simulink model "movementCueEast"  (R2012b)
settings: Solver=FixedStepDiscrete  SolverMode=SingleTasking  StartTime=0.0  StopTime=inf  RelTol=1e-3
model workspace (MAT data in the model file):
  Param = Simulink.Parameter
  Param.DataType = 'auto'
undefined symbols (not defined in the file or in its folder): blockNumber, expRandBinSize, expRandMax, expRandMin, expRandMu, holdDuration, macaddr, modelConstants, movementDuration, pause, randomSeed, repsPerBlock, restDuration, returnDuration, useRandomDelay, whichMovements
libraries: xpcethernetlib x13, Lib_FileLogger x9, xpcnetworkbufferlib x4, xpclib x3, dspmtrx3 x2, xpcparallelportlib x1, simulink x1, Lib_CerebusRead x1
settings Model: xpc_rtwmakecfg_data=_xpcetherlib__xpcether8255xlib__xpcetherGbElib__xpcnblib_  Creator=gilja  LastModifiedBy=NPTL
settings OptimizationCC: BlockReduction=off  InlineParams=on  InlineInvariantSignals=on  SimCompilerOptimization=On
settings HardwareCC: ProdIntDivRoundTo=Zero  ProdEndianess=LittleEndian  ProdHWDeviceType=Generic->32-bit x86 compatible
settings RTWCC: SystemTargetFile=xpctarget.tlc  TemplateMakefile=xpc_default_tmf  Description=xPC Target  ProcessScript=xpctarget_make_rtw_hook  RTWCompilerOptimization=On
settings CodeAppCC: MaxIdLength=62
settings xpcTargetCC: TargetFcnLib=ansi_tfl_table_tmw.mat  CodeReplacementLibrary=XPC_BLAS  ParMdlRefBuildCompliant=on  ConcurrentExecutionCompliant=on  CombineSignalStateStructs=off  GRTInterface=on  xPCTaskExecutionProfile=off  xPCRL32EventNumber=5000  RL32IRQSourceModifier=5  xPCIRQSourceBoard=Parallel_Port  xPCIOIRQSlot=0x378  xPCisDownloadable=off  xPCLoadParamSetFile=off  xPCConcurrentTasks=off  xPCEnableSFAnimation=off

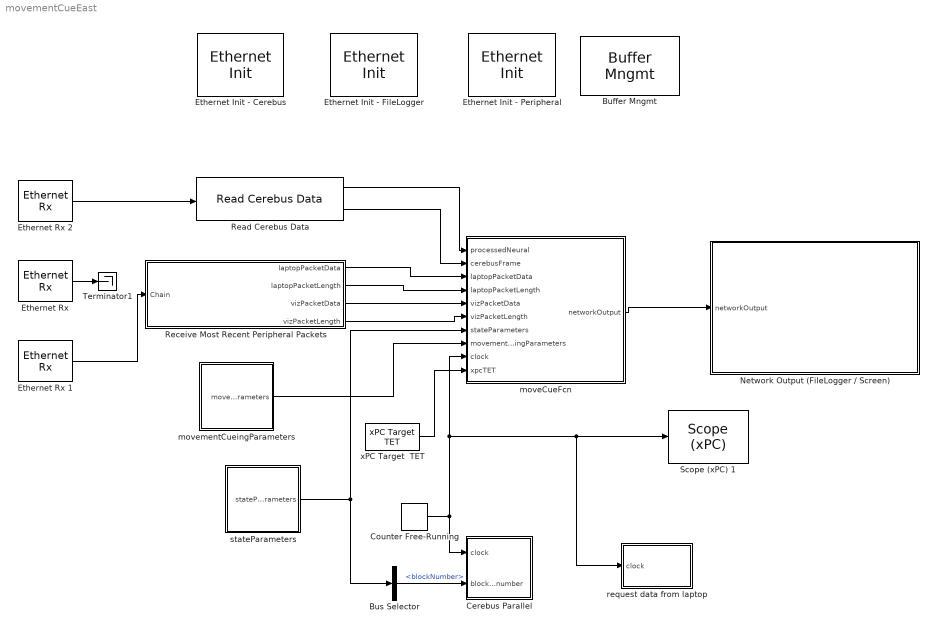
== system movementCueEast ==
  "Buffer Mngmt " : xpcnetworkbufferlib/Buffer Mngmt   Priority=-1  SampleTime=-1  PoolSizes=[100 10 10 200]  ShowTune=on
  Bus Selector : BusSelector  OutputSignals=blockNumber
  Cerebus Parallel : Subsystem
  Counter Free-Running : simulink/Sources/Counter Free-Running  NumBits=32  tsamp=-1
  Ethernet Init - Cerebus : xpcethernetlib/Ethernet Init   Priority=-1  ID=1  Driver=Intel Gigabit  Bus=3  Slot=14  SampleTime=-1  AddressSource=Specify  MAC=macaddr('00:00:00:00:00:00')  TxSA=off  RxPromiscuous=off  Multicast={}  RxBad=off  RxShort=off  MaxMTU=1518  TxThreshold=10  TxBuffers=128  RxBuffers=64  ShowTune=on  NumRxBlks=1
  Ethernet Init - FileLogger : xpcethernetlib/Ethernet Init   Priority=-1  ID=2  Driver=Intel Gigabit  Bus=3  Slot=13  SampleTime=-1  AddressSource=Specify  MAC=macaddr('00:00:00:00:00:00')  TxSA=off  RxPromiscuous=off  Multicast={}  RxBad=off  RxShort=off  MaxMTU=1518  TxThreshold=10  TxBuffers=128  RxBuffers=8  ShowTune=on  NumRxBlks=1
  Ethernet Init - Peripheral : xpcethernetlib/Ethernet Init   Priority=-1  ID=3  Driver=Intel Gigabit  Bus=2  Slot=0  SampleTime=-1  AddressSource=Specify  MAC=macaddr('00:00:00:00:00:00')  TxSA=off  RxPromiscuous=off  Multicast={}  RxBad=off  RxShort=off  MaxMTU=1518  TxThreshold=10  TxBuffers=128  RxBuffers=8  ShowTune=on  NumRxBlks=1
  "Ethernet Rx " : xpcethernetlib/Ethernet Rx   ID=2  SampleTime=modelConstants.sampleTime  Criteria=Receive all unmatched types [0 to 65535]  EtherType=[hex2dec('0000')]  BlkID=0
  Ethernet Rx 1 : xpcethernetlib/Ethernet Rx   ID=3  SampleTime=modelConstants.sampleTime  Criteria=Receive all unmatched types [0 to 65535]  EtherType=[hex2dec('0000')]  BlkID=0
  Ethernet Rx 2 : xpcethernetlib/Ethernet Rx   ID=1  SampleTime=modelConstants.sampleTime  Criteria=Receive all unmatched types [0 to 65535]  EtherType=[hex2dec('0000')]  BlkID=0
  Network Output (FileLogger / Screen) : Subsystem
  Read Cerebus Data : Lib_CerebusRead/Read Cerebus Data
  Receive Most Recent Peripheral Packets : Subsystem
  Scope (xPC) 1 : xpclib/Misc./Scope (xPC)   scopeno=1  scopetype=Target  autostart=on  viewmode=Numerical  formatstr='%15.6f'  grid=on  ylimits=[0,0]  nosamples=250  noprepostsamples=0  interleave=1  triggermode=FreeRun  triggersignal=1  triggerlevel=0.0  triggerslope=Either  triggerscope=1  triggersample=0  filename=data.dat  mode=Lazy  writesize=512  autorestart=off  dynamicfilemode=off  maxwritefilesize=512*1024^2
  Terminator1 : Terminator
  moveCueFcn : MATLAB Function  TreatAsAtomicUnit=on
  movementCueingParameters : Subsystem
  request data from laptop : Subsystem
  stateParameters : Subsystem
  "xPC Target  TET " : xpclib/Misc./xPC Target  TET   ts=0.001
  wires:
  Ethernet Rx 1/1 -> Receive Most Recent Peripheral Packets/1(Chain)
  moveCueFcn/1(networkOutput) -> Network Output (FileLogger / Screen)/1(networkOutput)
  stateParameters/1(stateParameters) -> Bus Selector/1, moveCueFcn/7(stateParameters)
  "Ethernet Rx "/1 -> Terminator1/1
  Counter Free-Running/1 -> Scope (xPC) 1/1, request data from laptop/1(clock), moveCueFcn/9(clock), Cerebus Parallel/1(clock)
  movementCueingParameters/1(movementCueingParameters) -> moveCueFcn/8(movementCueingParameters)
  Bus Selector/1 -> Cerebus Parallel/2(block number)  "<blockNumber>"
  Receive Most Recent Peripheral Packets/1(laptopPacketData) -> moveCueFcn/3(laptopPacketData)
  Receive Most Recent Peripheral Packets/2(laptopPacketLength) -> moveCueFcn/4(laptopPacketLength)
  Receive Most Recent Peripheral Packets/3(vizPacketData) -> moveCueFcn/5(vizPacketData)
  Receive Most Recent Peripheral Packets/4(vizPacketLength) -> moveCueFcn/6(vizPacketLength)
  Ethernet Rx 2/1 -> Read Cerebus Data/1
  Read Cerebus Data/1 -> moveCueFcn/1(processedNeural)
  Read Cerebus Data/2 -> moveCueFcn/2(cerebusFrame)
  "xPC Target  TET "/1 -> moveCueFcn/10(xpcTET)

== system movementCueEast/Cerebus Parallel ==
  clock : Inport
  block number : Inport  Port=2
  "Parallel Port DO " : xpcparallelportlib/Digital Output/Parallel Port DO   BaseMask=0x378  BaseString=0x378  Format=8 1-bit Channels  Channels=[1]  InitialValues=[0]  FinalActions=[0]  FinalValues=[0]  SampleTime=0.001  Mode=1
  cerebus Parallel : MATLAB Function  TreatAsAtomicUnit=on
  wires:
  block number/1 -> cerebus Parallel/2(blockNumber)
  clock/1 -> cerebus Parallel/1(clock)
  cerebus Parallel/1(digitalOut) -> "Parallel Port DO "/1

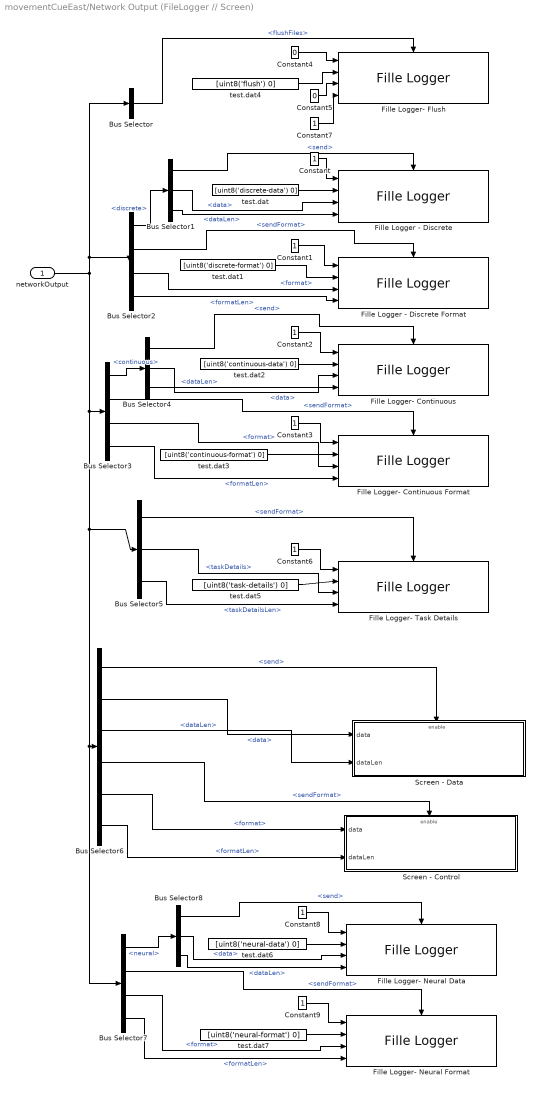
== system movementCueEast/Network Output (FileLogger // Screen) ==
  networkOutput : Inport  OutDataTypeStr=Bus: networkOutput
  Bus Selector : BusSelector  OutputSignals=flushFiles
  Bus Selector1 : BusSelector  OutputSignals=send,data,dataLen
  Bus Selector2 : BusSelector  OutputSignals=discrete,sendFormat,discrete.format,discrete.formatLen
  Bus Selector3 : BusSelector  OutputSignals=continuous,sendFormat,continuous.format,continuous.formatLen
  Bus Selector4 : BusSelector  OutputSignals=send,data,dataLen
  Bus Selector5 : BusSelector  OutputSignals=sendFormat,taskDetails,taskDetailsLen
  Bus Selector6 : BusSelector  OutputSignals=screen.send,screen.data,screen.dataLen,sendFormat,screen.format,screen.formatLen
  Bus Selector7 : BusSelector  OutputSignals=neural,sendFormat,neural.format,neural.formatLen
  Bus Selector8 : BusSelector  OutputSignals=send,data,dataLen
  Constant{,1..3,6,8..9} (7 alike) : Constant  OutDataTypeStr=boolean
  Constant4 : Constant  Value=0  OutDataTypeStr=boolean
  Constant5 : Constant  Value=0
  Constant7 : Constant  OutDataTypeStr=uint16
  Fille Logger - Discrete : Lib_FileLogger/Fille Logger
  "Fille Logger - Discrete Format " : Lib_FileLogger/Fille Logger
  Fille Logger- Continuous : Lib_FileLogger/Fille Logger
  Fille Logger- Continuous Format : Lib_FileLogger/Fille Logger
  Fille Logger- Flush : Lib_FileLogger/Fille Logger
  Fille Logger- Neural Data : Lib_FileLogger/Fille Logger
  Fille Logger- Neural Format : Lib_FileLogger/Fille Logger
  Fille Logger- Task Details : Lib_FileLogger/Fille Logger
  Screen - Control : Subsystem
  Screen - Data : Subsystem
  test.dat : Constant  Value=[uint8('discrete-data') 0]  OutDataTypeStr=uint8
  test.dat1 : Constant  Value=[uint8('discrete-format') 0]  OutDataTypeStr=uint8
  test.dat2 : Constant  Value=[uint8('continuous-data') 0]  OutDataTypeStr=uint8
  test.dat3 : Constant  Value=[uint8('continuous-format') 0]  OutDataTypeStr=uint8
  test.dat4 : Constant  Value=[uint8('flush') 0]  OutDataTypeStr=uint8
  test.dat5 : Constant  Value=[uint8('task-details') 0]  OutDataTypeStr=uint8
  test.dat6 : Constant  Value=[uint8('neural-data') 0]  OutDataTypeStr=uint8
  test.dat7 : Constant  Value=[uint8('neural-format') 0]  OutDataTypeStr=uint8
  wires:
  test.dat/1 -> Fille Logger - Discrete/2
  Constant1/1 -> "Fille Logger - Discrete Format "/1
  test.dat2/1 -> Fille Logger- Continuous/2
  test.dat1/1 -> "Fille Logger - Discrete Format "/2
  Constant2/1 -> Fille Logger- Continuous/1
  test.dat3/1 -> Fille Logger- Continuous Format/2
  Bus Selector3/2 -> Fille Logger- Continuous Format/Enable  "<sendFormat>"
  Bus Selector2/1 -> Bus Selector1/1  "<discrete>"
  Bus Selector1/1 -> Fille Logger - Discrete/Enable  "<send>"
  Constant/1 -> Fille Logger - Discrete/1
  Constant3/1 -> Fille Logger- Continuous Format/1
  Bus Selector4/2 -> Fille Logger- Continuous/3  "<data>"
  Bus Selector1/2 -> Fille Logger - Discrete/3  "<data>"
  Bus Selector2/2 -> "Fille Logger - Discrete Format "/Enable  "<sendFormat>"
  Constant4/1 -> Fille Logger- Flush/1
  test.dat4/1 -> Fille Logger- Flush/2
  Bus Selector3/3 -> Fille Logger- Continuous Format/3  "<format>"
  Bus Selector2/3 -> "Fille Logger - Discrete Format "/3  "<format>"
  Constant5/1 -> Fille Logger- Flush/3
  Bus Selector/1 -> Fille Logger- Flush/Enable  "<flushFiles>"
  networkOutput/1 -> Bus Selector2/1, Bus Selector/1, Bus Selector7/1, Bus Selector6/1, Bus Selector5/1, Bus Selector3/1
  Bus Selector4/1 -> Fille Logger- Continuous/Enable  "<send>"
  test.dat5/1 -> Fille Logger- Task Details/2
  Bus Selector5/1 -> Fille Logger- Task Details/Enable  "<sendFormat>"
  Constant6/1 -> Fille Logger- Task Details/1
  Bus Selector5/2 -> Fille Logger- Task Details/3  "<taskDetails>"
  Bus Selector6/1 -> Screen - Data/Enable  "<send>"
  Bus Selector6/2 -> Screen - Data/1(data)  "<data>"
  Bus Selector6/4 -> Screen - Control/Enable  "<sendFormat>"
  Bus Selector6/5 -> Screen - Control/1(data)  "<format>"
  Bus Selector1/3 -> Fille Logger - Discrete/4  "<dataLen>"
  Constant7/1 -> Fille Logger- Flush/4
  Bus Selector2/4 -> "Fille Logger - Discrete Format "/4  "<formatLen>"
  Bus Selector3/4 -> Fille Logger- Continuous Format/4  "<formatLen>"
  Bus Selector4/3 -> Fille Logger- Continuous/4  "<dataLen>"
  Bus Selector3/1 -> Bus Selector4/1  "<continuous>"
  Bus Selector5/3 -> Fille Logger- Task Details/4  "<taskDetailsLen>"
  Bus Selector6/3 -> Screen - Data/2(dataLen)  "<dataLen>"
  Bus Selector6/6 -> Screen - Control/2(dataLen)  "<formatLen>"
  test.dat6/1 -> Fille Logger- Neural Data/2
  Constant8/1 -> Fille Logger- Neural Data/1
  test.dat7/1 -> Fille Logger- Neural Format/2
  Bus Selector7/2 -> Fille Logger- Neural Format/Enable  "<sendFormat>"
  Bus Selector7/1 -> Bus Selector8/1  "<neural>"
  Constant9/1 -> Fille Logger- Neural Format/1
  Bus Selector8/2 -> Fille Logger- Neural Data/3  "<data>"
  Bus Selector7/3 -> Fille Logger- Neural Format/3  "<format>"
  Bus Selector8/1 -> Fille Logger- Neural Data/Enable  "<send>"
  Bus Selector7/4 -> Fille Logger- Neural Format/4  "<formatLen>"
  Bus Selector8/3 -> Fille Logger- Neural Data/4  "<dataLen>"

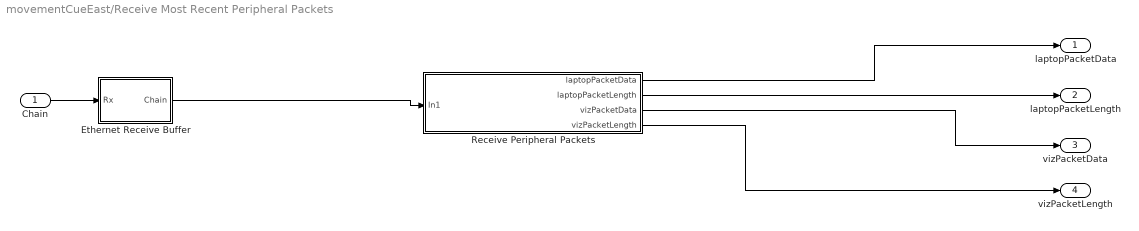
== system movementCueEast/Receive Most Recent Peripheral Packets ==
  Chain : Inport
  Ethernet Receive Buffer : Subsystem
  Receive Peripheral Packets : Subsystem
  laptopPacketData : Outport
  laptopPacketLength : Outport  Port=2
  vizPacketData : Outport  Port=3
  vizPacketLength : Outport  Port=4
  wires:
  Chain/1 -> Ethernet Receive Buffer/1(Rx)
  Ethernet Receive Buffer/1(Chain) -> Receive Peripheral Packets/1(In1)
  Receive Peripheral Packets/1(laptopPacketData) -> laptopPacketData/1
  Receive Peripheral Packets/2(laptopPacketLength) -> laptopPacketLength/1
  Receive Peripheral Packets/3(vizPacketData) -> vizPacketData/1
  Receive Peripheral Packets/4(vizPacketLength) -> vizPacketLength/1

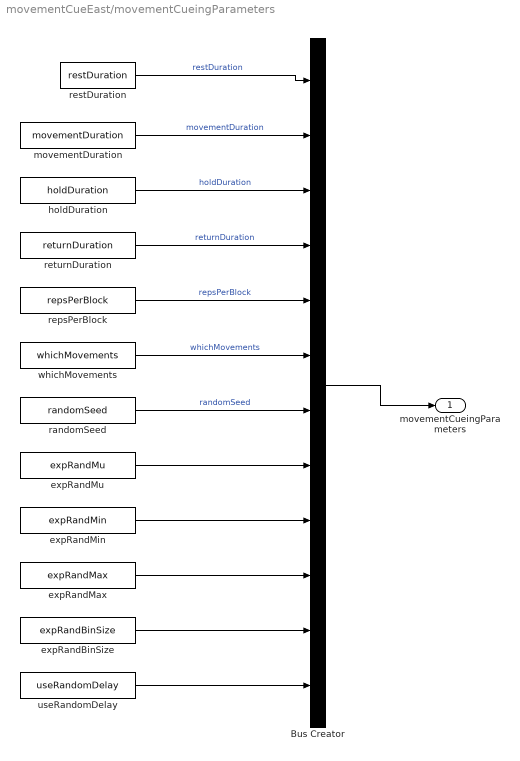
== system movementCueEast/movementCueingParameters ==
  Bus Creator : BusCreator  Inputs=12  OutDataTypeStr=Bus: movementParams  NonVirtualBus=on
  expRandBinSize : Constant  Value=expRandBinSize
  expRandMax : Constant  Value=expRandMax
  expRandMin : Constant  Value=expRandMin
  expRandMu : Constant  Value=expRandMu
  holdDuration : Constant  Value=holdDuration
  movementDuration : Constant  Value=movementDuration
  randomSeed : Constant  Value=randomSeed
  repsPerBlock : Constant  Value=repsPerBlock
  restDuration : Constant  Value=restDuration
  returnDuration : Constant  Value=returnDuration
  useRandomDelay : Constant  Value=useRandomDelay
  whichMovements : Constant  Value=whichMovements
  movementCueingParameters : Outport
  wires:
  restDuration/1 -> Bus Creator/1  "restDuration"
  Bus Creator/1 -> movementCueingParameters/1
  movementDuration/1 -> Bus Creator/2  "movementDuration"
  holdDuration/1 -> Bus Creator/3  "holdDuration"
  returnDuration/1 -> Bus Creator/4  "returnDuration"
  repsPerBlock/1 -> Bus Creator/5  "repsPerBlock"
  useRandomDelay/1 -> Bus Creator/12
  expRandBinSize/1 -> Bus Creator/11
  expRandMax/1 -> Bus Creator/10
  expRandMin/1 -> Bus Creator/9
  expRandMu/1 -> Bus Creator/8
  randomSeed/1 -> Bus Creator/7  "randomSeed"
  whichMovements/1 -> Bus Creator/6  "whichMovements"

== system movementCueEast/request data from laptop ==
  clock : Inport
  Laptop Data Request : MATLAB Function  TreatAsAtomicUnit=on
  UDP to Laptop : Subsystem
  wires:
  Laptop Data Request/3(dataLen) -> UDP to Laptop/2(udpDataLen)
  Laptop Data Request/2(data) -> UDP to Laptop/1(udpData)
  Laptop Data Request/1(send) -> UDP to Laptop/Enable
  clock/1 -> Laptop Data Request/1(clock)

== system movementCueEast/stateParameters ==
  Bus Creator : BusCreator  Inputs='pause','blockNumber'  OutDataTypeStr=Bus: stateParams  NonVirtualBus=on
  blockNumber : Constant  Value=blockNumber  OutDataTypeStr=uint32
  pause : Constant  Value=pause  OutDataTypeStr=boolean
  stateParameters : Outport
  wires:
  pause/1 -> Bus Creator/1  "pause"
  Bus Creator/1 -> stateParameters/1
  blockNumber/1 -> Bus Creator/2  "blockNumber"

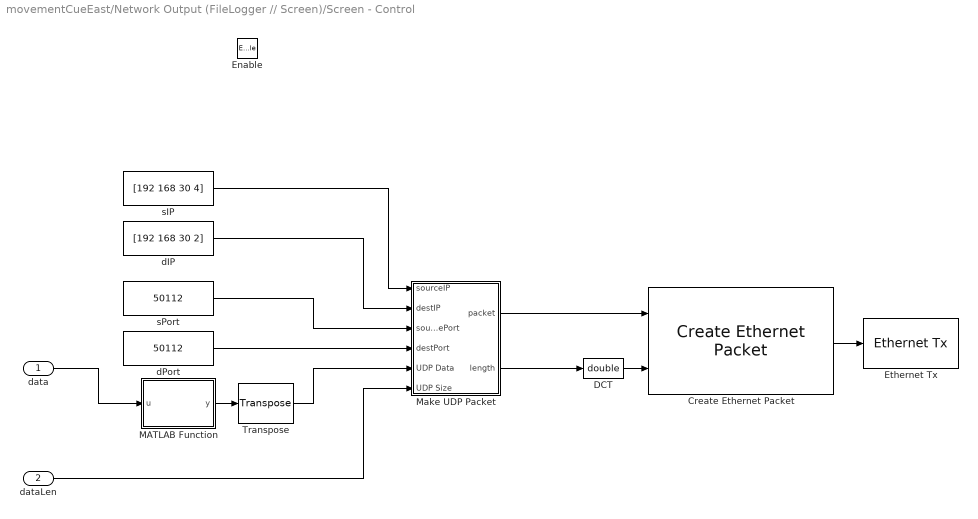
== system movementCueEast/Network Output (FileLogger // Screen)/Screen - Control ==
  data : Inport
  dataLen : Inport  Port=2
  Enable : EnablePort
  "Create Ethernet Packet " : xpcethernetlib/Create Ethernet Packet   DstMac=macaddr('FF:FF:FF:FF:FF:FF')  EtherType=hex2dec('0800')
  DCT : DataTypeConversion  OutDataTypeStr=double
  "Ethernet Tx " : xpcethernetlib/Ethernet Tx   ID=3  SampleTime=-1
  MATLAB Function : MATLAB Function  TreatAsAtomicUnit=on
  Make UDP Packet : Subsystem
  Transpose : dspmtrx3/Transpose  Hermitian=off  overflowFlag=off
  dIP : Constant  Value=[192 168 30 2]  OutDataTypeStr=uint8
  dPort : Constant  Value=50112  OutDataTypeStr=uint16
  sIP : Constant  Value=[192 168 30 4]  OutDataTypeStr=uint8
  sPort : Constant  Value=50112  OutDataTypeStr=uint16
  wires:
  dPort/1 -> Make UDP Packet/4(destPort)
  Make UDP Packet/2(length) -> DCT/1
  "Create Ethernet Packet "/1 -> "Ethernet Tx "/1
  Make UDP Packet/1(packet) -> "Create Ethernet Packet "/1
  DCT/1 -> "Create Ethernet Packet "/2
  data/1 -> MATLAB Function/1(u)
  MATLAB Function/1(y) -> Transpose/1
  dataLen/1 -> Make UDP Packet/6(UDP Size)
  sPort/1 -> Make UDP Packet/3(sourcePort)
  dIP/1 -> Make UDP Packet/2(destIP)
  sIP/1 -> Make UDP Packet/1(sourceIP)
  Transpose/1 -> Make UDP Packet/5(UDP Data)

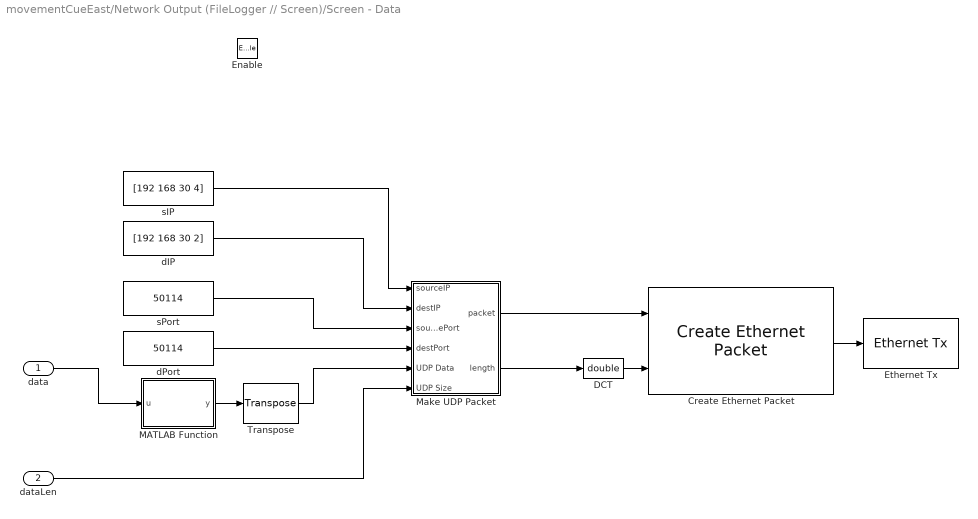
== system movementCueEast/Network Output (FileLogger // Screen)/Screen - Data ==
  data : Inport
  dataLen : Inport  Port=2
  Enable : EnablePort
  "Create Ethernet Packet " : xpcethernetlib/Create Ethernet Packet   DstMac=macaddr('FF:FF:FF:FF:FF:FF')  EtherType=hex2dec('0800')
  DCT : DataTypeConversion  OutDataTypeStr=double
  "Ethernet Tx " : xpcethernetlib/Ethernet Tx   ID=3  SampleTime=-1
  MATLAB Function : MATLAB Function  TreatAsAtomicUnit=on
  Make UDP Packet : Subsystem
  Transpose : dspmtrx3/Transpose  Hermitian=off  overflowFlag=off
  dIP : Constant  Value=[192 168 30 2]  OutDataTypeStr=uint8
  dPort : Constant  Value=50114  OutDataTypeStr=uint16
  sIP : Constant  Value=[192 168 30 4]  OutDataTypeStr=uint8
  sPort : Constant  Value=50114  OutDataTypeStr=uint16
  wires:
  dPort/1 -> Make UDP Packet/4(destPort)
  Make UDP Packet/2(length) -> DCT/1
  "Create Ethernet Packet "/1 -> "Ethernet Tx "/1
  Make UDP Packet/1(packet) -> "Create Ethernet Packet "/1
  DCT/1 -> "Create Ethernet Packet "/2
  data/1 -> MATLAB Function/1(u)
  MATLAB Function/1(y) -> Transpose/1
  dataLen/1 -> Make UDP Packet/6(UDP Size)
  sPort/1 -> Make UDP Packet/3(sourcePort)
  dIP/1 -> Make UDP Packet/2(destIP)
  sIP/1 -> Make UDP Packet/1(sourceIP)
  Transpose/1 -> Make UDP Packet/5(UDP Data)

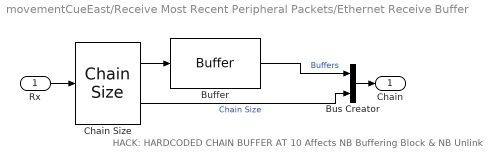
== system movementCueEast/Receive Most Recent Peripheral Packets/Ethernet Receive Buffer ==
  note: HACK: HARDCODED CHAIN BUFFER AT 10
      | Affects NB Buffering Block & NB Unlink
  Rx : Inport
  Buffer : xpcnetworkbufferlib/Buffer   ChainSize=10  BufferSize=0  Threshold=0
  Bus Creator : BusCreator  Inputs=2
  "Chain Size " : xpcnetworkbufferlib/Chain Size 
  Chain : Outport
  wires:
  Buffer/1 -> Bus Creator/1  "Buffers"
  Bus Creator/1 -> Chain/1
  "Chain Size "/2 -> Bus Creator/2  "Chain Size"
  Rx/1 -> "Chain Size "/1
  "Chain Size "/1 -> Buffer/1

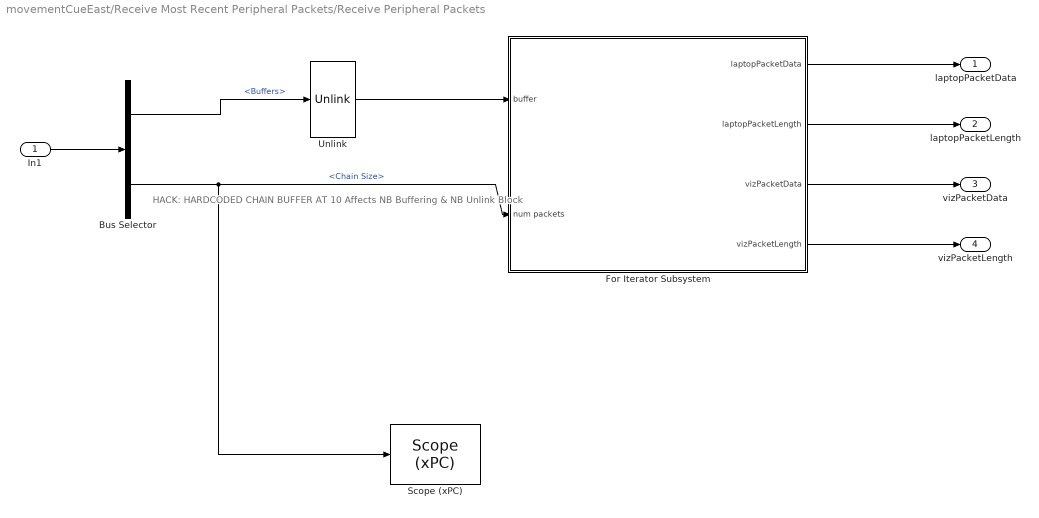
== system movementCueEast/Receive Most Recent Peripheral Packets/Receive Peripheral Packets ==
  note: HACK: HARDCODED CHAIN BUFFER AT 10
      | Affects NB Buffering & NB Unlink Block
  In1 : Inport
  Bus Selector : BusSelector  OutputSignals=Buffers,Chain Size
  For Iterator Subsystem : Subsystem  TreatAsAtomicUnit=on
  "Scope (xPC) " : xpclib/Misc./Scope (xPC)   scopeno=3  scopetype=Target  autostart=on  viewmode=Numerical  formatstr='%15.6f'  grid=on  ylimits=[0,0]  nosamples=250  noprepostsamples=0  interleave=1  triggermode=FreeRun  triggersignal=1  triggerlevel=0.0  triggerslope=Either  triggerscope=1  triggersample=0  filename=data.dat  mode=Lazy  writesize=512  autorestart=off  dynamicfilemode=off  maxwritefilesize=512*1024^2
  "Unlink " : xpcnetworkbufferlib/Unlink   VectorLength=10
  laptopPacketData : Outport
  laptopPacketLength : Outport  Port=2
  vizPacketData : Outport  Port=3
  vizPacketLength : Outport  Port=4
  wires:
  Bus Selector/1 -> "Unlink "/1  "<Buffers>"
  "Unlink "/1 -> For Iterator Subsystem/1(buffer)
  Bus Selector/2 -> "Scope (xPC) "/1, For Iterator Subsystem/2(num packets)  "<Chain Size>"
  In1/1 -> Bus Selector/1
  For Iterator Subsystem/1(laptopPacketData) -> laptopPacketData/1
  For Iterator Subsystem/2(laptopPacketLength) -> laptopPacketLength/1
  For Iterator Subsystem/3(vizPacketData) -> vizPacketData/1
  For Iterator Subsystem/4(vizPacketLength) -> vizPacketLength/1

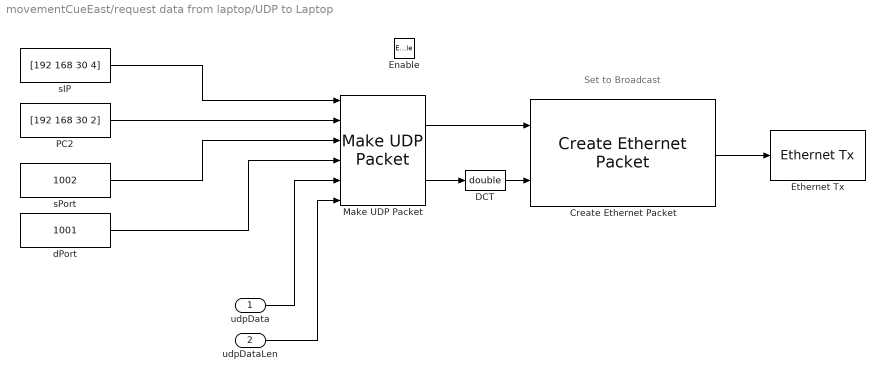
== system movementCueEast/request data from laptop/UDP to Laptop ==
  note: Set to Broadcast
  udpData : Inport
  udpDataLen : Inport  Port=2
  Enable : EnablePort
  "Create Ethernet Packet " : xpcethernetlib/Create Ethernet Packet   DstMac=macaddr('FF:FF:FF:FF:FF:FF')  EtherType=hex2dec('0800')
  DCT : DataTypeConversion  OutDataTypeStr=double
  "Ethernet Tx " : xpcethernetlib/Ethernet Tx   ID=3  SampleTime=-1
  Make UDP Packet : Lib_FileLogger/Fille Logger/Make UDP Packet
  PC2 : Constant  Value=[192 168 30 2]  OutDataTypeStr=uint8
  dPort : Constant  Value=1001  OutDataTypeStr=uint16
  sIP : Constant  Value=[192 168 30 4]  OutDataTypeStr=uint8
  sPort : Constant  Value=1002  OutDataTypeStr=uint16
  wires:
  dPort/1 -> Make UDP Packet/4
  sIP/1 -> Make UDP Packet/1
  Make UDP Packet/2 -> DCT/1
  Make UDP Packet/1 -> "Create Ethernet Packet "/1
  DCT/1 -> "Create Ethernet Packet "/2
  PC2/1 -> Make UDP Packet/2
  sPort/1 -> Make UDP Packet/3
  udpDataLen/1 -> Make UDP Packet/6
  "Create Ethernet Packet "/1 -> "Ethernet Tx "/1
  udpData/1 -> Make UDP Packet/5

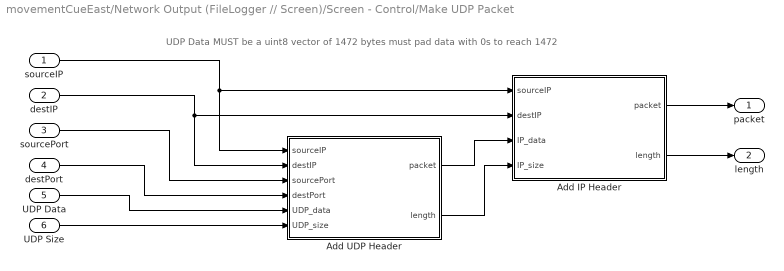
== system movementCueEast/Network Output (FileLogger // Screen)/Screen - Control/Make UDP Packet ==
  note: UDP Data MUST be a uint8 vector of 1472 bytes
      | must pad data with 0s to reach 1472
  sourceIP : Inport
  destIP : Inport  Port=2
  sourcePort : Inport  Port=3
  destPort : Inport  Port=4
  UDP Data : Inport  Port=5
  UDP Size : Inport  Port=6
  Add IP Header : MATLAB Function  TreatAsAtomicUnit=on
  Add UDP Header : MATLAB Function  TreatAsAtomicUnit=on
  packet : Outport
  length : Outport  Port=2
  wires:
  Add UDP Header/2(length) -> Add IP Header/4(IP_size)
  Add UDP Header/1(packet) -> Add IP Header/3(IP_data)
  sourceIP/1 -> Add UDP Header/1(sourceIP), Add IP Header/1(sourceIP)
  destIP/1 -> Add UDP Header/2(destIP), Add IP Header/2(destIP)
  sourcePort/1 -> Add UDP Header/3(sourcePort)
  destPort/1 -> Add UDP Header/4(destPort)
  UDP Data/1 -> Add UDP Header/5(UDP_data)
  Add IP Header/1(packet) -> packet/1
  Add IP Header/2(length) -> length/1
  UDP Size/1 -> Add UDP Header/6(UDP_size)

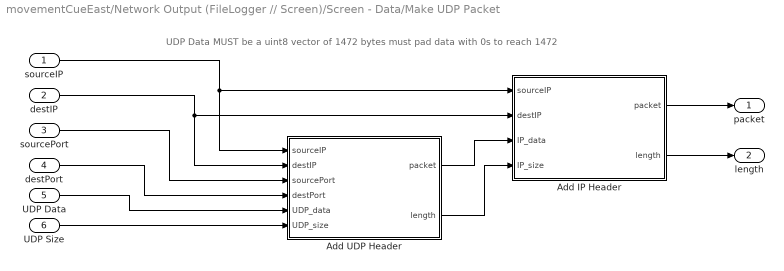
== system movementCueEast/Network Output (FileLogger // Screen)/Screen - Data/Make UDP Packet ==
  note: UDP Data MUST be a uint8 vector of 1472 bytes
      | must pad data with 0s to reach 1472
  sourceIP : Inport
  destIP : Inport  Port=2
  sourcePort : Inport  Port=3
  destPort : Inport  Port=4
  UDP Data : Inport  Port=5
  UDP Size : Inport  Port=6
  Add IP Header : MATLAB Function  TreatAsAtomicUnit=on
  Add UDP Header : MATLAB Function  TreatAsAtomicUnit=on
  packet : Outport
  length : Outport  Port=2
  wires:
  Add UDP Header/2(length) -> Add IP Header/4(IP_size)
  Add UDP Header/1(packet) -> Add IP Header/3(IP_data)
  sourceIP/1 -> Add UDP Header/1(sourceIP), Add IP Header/1(sourceIP)
  destIP/1 -> Add UDP Header/2(destIP), Add IP Header/2(destIP)
  sourcePort/1 -> Add UDP Header/3(sourcePort)
  destPort/1 -> Add UDP Header/4(destPort)
  UDP Data/1 -> Add UDP Header/5(UDP_data)
  Add IP Header/1(packet) -> packet/1
  Add IP Header/2(length) -> length/1
  UDP Size/1 -> Add UDP Header/6(UDP_size)

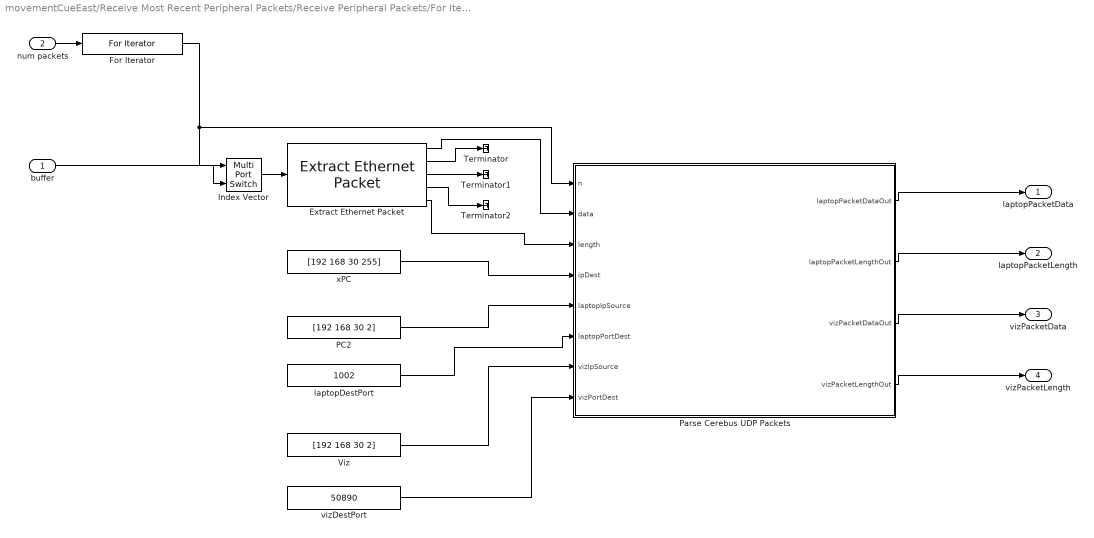
== system movementCueEast/Receive Most Recent Peripheral Packets/Receive Peripheral Packets/For Iterator Subsystem ==
  buffer : Inport
  num packets : Inport  Port=2
  Extract Ethernet Packet : xpcethernetlib/Extract Ethernet Packet   EthernetDataSize=1500
  For Iterator : ForIterator  IterationSource=external  IterationVariableDataType=int8
  Index Vector : MultiPortSwitch  Inputs=1
  PC2 : Constant  Value=[192 168 30 2]  OutDataTypeStr=uint8
  Parse Cerebus UDP Packets : MATLAB Function  TreatAsAtomicUnit=on
  Terminator : Terminator
  Terminator1 : Terminator
  Terminator2 : Terminator
  Viz : Constant  Value=[192 168 30 2]  OutDataTypeStr=uint8
  laptopDestPort : Constant  Value=1002  OutDataTypeStr=uint16
  vizDestPort : Constant  Value=50890  OutDataTypeStr=uint16
  xPC : Constant  Value=[192 168 30 255]  OutDataTypeStr=uint8
  laptopPacketData : Outport  OutDataTypeStr=uint8  PortDimensions=1500
  laptopPacketLength : Outport  Port=2
  vizPacketData : Outport  Port=3  OutDataTypeStr=uint8  PortDimensions=1500
  vizPacketLength : Outport  Port=4
  wires:
  For Iterator/1 -> Parse Cerebus UDP Packets/1(n), Index Vector/1
  Extract Ethernet Packet/5 -> Parse Cerebus UDP Packets/3(length)
  num packets/1 -> For Iterator/1
  buffer/1 -> Index Vector/2
  Index Vector/1 -> Extract Ethernet Packet/1
  Extract Ethernet Packet/1 -> Parse Cerebus UDP Packets/2(data)
  Extract Ethernet Packet/2 -> Terminator/1
  Extract Ethernet Packet/3 -> Terminator1/1
  Extract Ethernet Packet/4 -> Terminator2/1
  PC2/1 -> Parse Cerebus UDP Packets/5(laptopIpSource)
  xPC/1 -> Parse Cerebus UDP Packets/4(ipDest)
  laptopDestPort/1 -> Parse Cerebus UDP Packets/6(laptopPortDest)
  Parse Cerebus UDP Packets/1(laptopPacketDataOut) -> laptopPacketData/1
  Parse Cerebus UDP Packets/2(laptopPacketLengthOut) -> laptopPacketLength/1
  Parse Cerebus UDP Packets/3(vizPacketDataOut) -> vizPacketData/1
  Parse Cerebus UDP Packets/4(vizPacketLengthOut) -> vizPacketLength/1
  Viz/1 -> Parse Cerebus UDP Packets/7(vizIpSource)
  vizDestPort/1 -> Parse Cerebus UDP Packets/8(vizPortDest)

== matlab function movementCueEast/Network Output (FileLogger // Screen)/Screen - Data/Make UDP Packet/Add UDP Header ==
  data: sourceIP input uint8 size=[1 4]; packet output; destIP input uint8 size=[1 4]; sourcePort input uint16 size=[1 1]; destPort input uint16 size=[1 1]; UDP_data input uint8; UDP_size input uint16 size=[1 1]; length output uint16 size=[1 1]
function [packet, length] = makeUDP(sourceIP, destIP, sourcePort, destPort, UDP_data, UDP_size)
% create UDP packet

% sourceIP and destIP are 1x4 uint8 of the IP (in address order)
% sourcePort and destPort are uint16
% UDP_data is uint8 of 1xN packet data
% UDP_size is uint16 size of UDP_data
%
% NOTE: UDP_size MUST BE EVEN
FFFF = uint16(hex2dec('FFFF'));

protocol = uint8(hex2dec('11'));

length = UDP_size + uint16(8);

length_BE = (typecast(length, 'uint8')); % flip to big endian
length_BE = length_BE(end:-1:1);

sourcePort_BE = (typecast(sourcePort, 'uint8'));
sourcePort_BE = sourcePort_BE(end:-1:1);

destPort_BE   = (typecast(destPort,   'uint8'));
destPort_BE = destPort_BE(end:-1:1);

header = [sourcePort_BE destPort_BE length_BE uint8([0 0])];

pseudoHeader = [sourceIP destIP uint8(0) protocol length_BE];

% header(7:8) = typecast( bitcmp(uint16(sum( typecast(bitcmp([pseudoHeader header UDP_data]), 'uint16') ))), 'uint8');


checksum = FFFF - uint16(mod( uint32(sum( typecast([pseudoHeader header UDP_data], 'uint16') )), uint32(FFFF) ));
header(7:8) = typecast(checksum, 'uint8');

packet = [ header UDP_data ];

== matlab function movementCueEast/Network Output (FileLogger // Screen)/Screen - Data/Make UDP Packet/Add IP Header ==
  data: sourceIP input uint8 size=[1 4]; packet output uint8; destIP input uint8 size=[1 4]; IP_data input uint8; IP_size input uint16 size=[1 1]; length output uint16 size=[1 1]
function [packet, length] = makeIP(sourceIP, destIP, IP_data, IP_size)
% create IP packet

FFFF = uint16(hex2dec('FFFF'));

version_IHL = uint8(69); % IPv4 and IP header length of 5
ToS = uint8(0); % no QOS on network

length = IP_size + uint16(20); % hardcode header length to 5

length_BE = (typecast(length, 'uint8')); % change to big endian
length_BE = length_BE(end:-1:1);

% counter
persistent ID % identification
if isempty(ID)
    ID = uint16(0);
else
    ID = ID + 1;
end

ff = [ uint8(bin2dec('01000000')) 0 ]; % don't fragment packets

TTL = uint8(10); % ttl to 10 seconds/hops

protocol = uint8(hex2dec('11')); % UDP Protocol


header = [ version_IHL ToS length_BE typecast(ID, 'uint8') ff TTL protocol 0 0 sourceIP destIP];

% header(11:12) = typecast(bitcmp(uint16(sum( typecast(bitcmp(header), 'uint16') ))), 'uint8'); % checksum

checksum = FFFF - uint16(mod( uint32(sum( typecast(header, 'uint16') )), uint32(FFFF) ));
header(11:12) = typecast(checksum, 'uint8');

packet = [ header IP_data ];

== matlab function movementCueEast/Network Output (FileLogger // Screen)/Screen - Data/MATLAB Function ==
  data: u input; y output
function y = padData(u)

z = uint8(zeros(1434, 1))';

z(1:length(u)) = u;

y = z';

== matlab function movementCueEast/Network Output (FileLogger // Screen)/Screen - Control/MATLAB Function ==
  data: u input; y output
function y = padData(u)

z = uint8(zeros(1434, 1))';

z(1:length(u)) = u;

y = z';

== matlab function movementCueEast/Network Output (FileLogger // Screen)/Screen - Control/Make UDP Packet/Add IP Header ==
  data: sourceIP input uint8 size=[1 4]; packet output uint8; destIP input uint8 size=[1 4]; IP_data input uint8; IP_size input uint16 size=[1 1]; length output uint16 size=[1 1]
function [packet, length] = makeIP(sourceIP, destIP, IP_data, IP_size)
% create IP packet

FFFF = uint16(hex2dec('FFFF'));

version_IHL = uint8(69); % IPv4 and IP header length of 5
ToS = uint8(0); % no QOS on network

length = IP_size + uint16(20); % hardcode header length to 5

length_BE = (typecast(length, 'uint8')); % change to big endian
length_BE = length_BE(end:-1:1);

% counter
persistent ID % identification
if isempty(ID)
    ID = uint16(0);
else
    ID = ID + 1;
end

ff = [ uint8(bin2dec('01000000')) 0 ]; % don't fragment packets

TTL = uint8(10); % ttl to 10 seconds/hops

protocol = uint8(hex2dec('11')); % UDP Protocol


header = [ version_IHL ToS length_BE typecast(ID, 'uint8') ff TTL protocol 0 0 sourceIP destIP];

% header(11:12) = typecast(bitcmp(uint16(sum( typecast(bitcmp(header), 'uint16') ))), 'uint8'); % checksum

checksum = FFFF - uint16(mod( uint32(sum( typecast(header, 'uint16') )), uint32(FFFF) ));
header(11:12) = typecast(checksum, 'uint8');

packet = [ header IP_data ];

== matlab function movementCueEast/Network Output (FileLogger // Screen)/Screen - Control/Make UDP Packet/Add UDP Header ==
  data: sourceIP input uint8 size=[1 4]; packet output; destIP input uint8 size=[1 4]; sourcePort input uint16 size=[1 1]; destPort input uint16 size=[1 1]; UDP_data input uint8; UDP_size input uint16 size=[1 1]; length output uint16 size=[1 1]
function [packet, length] = makeUDP(sourceIP, destIP, sourcePort, destPort, UDP_data, UDP_size)
% create UDP packet

% sourceIP and destIP are 1x4 uint8 of the IP (in address order)
% sourcePort and destPort are uint16
% UDP_data is uint8 of 1xN packet data
% UDP_size is uint16 size of UDP_data
%
% NOTE: UDP_size MUST BE EVEN
FFFF = uint16(hex2dec('FFFF'));

protocol = uint8(hex2dec('11'));

length = UDP_size + uint16(8);

length_BE = (typecast(length, 'uint8')); % flip to big endian
length_BE = length_BE(end:-1:1);

sourcePort_BE = (typecast(sourcePort, 'uint8'));
sourcePort_BE = sourcePort_BE(end:-1:1);

destPort_BE   = (typecast(destPort,   'uint8'));
destPort_BE = destPort_BE(end:-1:1);

header = [sourcePort_BE destPort_BE length_BE uint8([0 0])];

pseudoHeader = [sourceIP destIP uint8(0) protocol length_BE];

% header(7:8) = typecast( bitcmp(uint16(sum( typecast(bitcmp([pseudoHeader header UDP_data]), 'uint16') ))), 'uint8');


checksum = FFFF - uint16(mod( uint32(sum( typecast([pseudoHeader header UDP_data], 'uint16') )), uint32(FFFF) ));
header(7:8) = typecast(checksum, 'uint8');

packet = [ header UDP_data ];

== matlab function movementCueEast/Receive Most Recent Peripheral Packets/Receive Peripheral Packets/For Iterator Subsystem/Parse Cerebus UDP Packets ==
  data: laptopPacketDataOut output; laptopPacketLengthOut output; n input; data input uint8; vizPacketDataOut output; length input; ipDest input; laptopIpSource input; laptopPortDest input; vizPacketLengthOut output; vizIpSource input; vizPortDest input
function [laptopPacketDataOut, laptopPacketLengthOut, vizPacketDataOut, vizPacketLengthOut]  = parsePacketFromIP(n, data, length, ipDest, laptopIpSource, laptopPortDest, vizIpSource, vizPortDest)
%#codegen 

%%%%%%%%%%%%%%%%%%%%%%%%%%%%%
%
% parse for specific ip address
%
% Vikash 
% NPTL 
% Stanford University 
%
%%%%%%%%%%%%%%%%%%%%%%%%%%%%%

%%%%%%%%%%%%%%%%%%%%%%%%%%%%%
%
% Outputs:
%
% packetData - data from first packet to match this IP
% packetLength - length of the matching packet data
% 
%%%%%%%%%%%%%%%%%%%%%%%%%%%%%

persistent packetFound packetData packetLength;

if(isempty(packetFound))
    laptopPacketFound = false;
    laptopPacketData = coder.nullcopy(uint8(zeros(1500, 1)));
    laptopPacketLength = 0;
    vizPacketFound = false;
    vizPacketData = coder.nullcopy(uint8(zeros(1500, 1)));
    vizPacketLength = 0;
end

if(n == 1) % First loop for this tick, can't combine with persistent declarations
    laptopPacketFound = false;
    laptopPacketData = coder.nullcopy(uint8(zeros(1500, 1)));
    laptopPacketLength = 0;
    vizPacketFound = false;
    vizPacketData = coder.nullcopy(uint8(zeros(1500, 1)));
    vizPacketLength = 0;
end

if(~laptopPacketFound)
    if(all(data(13:16) == laptopIpSource) ...
            && all(data(17:20) == ipDest) ...
            && all(laptopPortDest == typecast(data(24:-1:23), 'uint16')))
        laptopPacketFound = true;
        laptopPacketData = data;
        laptopPacketLength = length;
    end
end

if(~vizPacketFound)
    if(all(data(13:16) == vizIpSource) ...
            && all(data(17:20) == ipDest) ...
            && all(vizPortDest == typecast(data(24:-1:23), 'uint16')))
        vizPacketFound = true;
        vizPacketData = data;
        vizPacketLength = length;
    end
end

laptopPacketDataOut = laptopPacketData;
laptopPacketLengthOut = laptopPacketLength;

vizPacketDataOut = vizPacketData;
vizPacketLengthOut = vizPacketLength;

== matlab function movementCueEast/moveCueFcn ==
  data: processedNeural input; cerebusFrame input; laptopPacketData input uint8 size=1500; networkOutput output Bus: networkOutput; laptopPacketLength input size=1; vizPacketData input; vizPacketLength input; stateParameters input Bus: stateParams size=1; movementCueingParameters input Bus: movementParams; clock input; xpcTET input
function networkOutput  = movementCueingTask(processedNeural, cerebusFrame, laptopPacketData, laptopPacketLength, vizPacketData, vizPacketLength, stateParameters, movementCueingParameters, clock, xpcTET)
%function networkOutput  = movementCueingTask(packetData, packetLength, pause, mouseOn, clock)
%#codegen


%% CONSTANTS
TASK_NAME = 'movementCue';
VERSION_ID = single(2.003);
blockNumber = uint32(0); % Place holder, to be updated for cerebus sync

MAX_REPETITIONS = 200; %% just used to bound memory usage, increase if we'll ever do larger blocks

% %% STATE MACHINE CONSTANTS
% STATE_INIT = uint32(0);
% STATE_MOVEMENT_TEXT = uint32(1);
% STATE_GO_CUE = uint32(2);
% STATE_HOLD_CUE = uint32(3);
% STATE_RETURN_CUE = uint32(4);
% STATE_REST_CUE = uint32(5);
% STATE_END = uint32(6);


%% TASK DETAILS PACKET
formatAndPacket.data = uint8(zeros(1,1400));
formatAndPacket.dataLen = uint16(0);
formatAndPacket.format = uint8(zeros(1,1400));
formatAndPacket.formatLen = uint16(0);
formatAndPacket.send = false;
networkOutput.flushFiles = false; 
[networkOutput.taskDetails networkOutput.taskDetailsLen] = packTaskDetails(TASK_NAME, VERSION_ID, ...
    'STATE_INIT', uint32(MovementStates.STATE_INIT), ...
    'STATE_PRE_MOVE', uint32(MovementStates.STATE_PRE_MOVE), ...
    'STATE_MOVEMENT_TEXT', uint32(MovementStates.STATE_MOVEMENT_TEXT),...
    'STATE_GO_CUE', uint32(MovementStates.STATE_GO_CUE), ...
    'STATE_HOLD_CUE', uint32(MovementStates.STATE_HOLD_CUE), ...
    'STATE_RETURN_CUE', uint32(MovementStates.STATE_RETURN_CUE), ...
    'STATE_REST_CUE', uint32(MovementStates.STATE_REST_CUE),...
    'STATE_END', uint32(MovementStates.STATE_END),...
    'MOVE_FIST', uint32(movementTypes.FIST),...
    'MOVE_THUMB', uint32(movementTypes.THUMB),...
    'MOVE_INDEX', uint32(movementTypes.INDEX),...
    'MOVE_MIDDLE', uint32(movementTypes.MIDDLE),...
    'MOVE_RING', uint32(movementTypes.RING),...
    'MOVE_WRISTFLEX', uint32(movementTypes.WRISTFLEX),...
    'MOVE_WRISTROT', uint32(movementTypes.WRISTROT),...
    'MOVE_ELBOWFLEX', uint32(movementTypes.ELBOWFLEX),...
    'MOVE_HUMERALIN', uint32(movementTypes.HUMERALIN),...
    'MOVE_ULNAR', uint32(movementTypes.ULNAR)...
);
networkOutput.discrete = formatAndPacket;
networkOutput.continuous = formatAndPacket;
networkOutput.screen = formatAndPacket;
networkOutput.sound = formatAndPacket;
networkOutput.sendFormat = false;
networkOutput.neural = formatAndPacket;


%% DEFINE PERSISTENTS
persistent state behaviorPacket vizPacket;
persistent pauseTriggered;
persistent stateTimer;
persistent movementText;
persistent delayPeriodDuration movementDuration holdDuration restDuration returnDuration randomSeed repsPerBlock whichMovements;
persistent movementOrder numMovements movementInds;
persistent orderSet;
persistent expRandMu expRandMin expRandMax expRandBinSize useRandomDelay;
persistent cycleNum;
persistent movementNum;
persistent currentMovement;

%% INITIALIZE PERSISTENTS
if(isempty(state))
    state = uint16(MovementStates.STATE_INIT);
    behaviorPacket = initBehaviorPacket;
    vizPacket = initVizPacket;
    stateTimer = 0;
    movementText = char(zeros([1 50]));
    pauseTriggered = true;
    
    %% buffer all the parameters off the bus
    movementDuration = movementCueingParameters.movementDuration;
    holdDuration = movementCueingParameters.holdDuration;
    restDuration = movementCueingParameters.restDuration;
    returnDuration = movementCueingParameters.returnDuration;
    repsPerBlock = movementCueingParameters.repsPerBlock;
    randomSeed = movementCueingParameters.randomSeed;
    whichMovements = movementCueingParameters.whichMovements;

    useRandomDelay = movementCueingParameters.useRandomDelay;    
    expRandMu = movementCueingParameters.expRandMu;
    expRandMin = movementCueingParameters.expRandMin;
    expRandMax = movementCueingParameters.expRandMax;
    expRandBinSize = movementCueingParameters.expRandBinSize;
    delayPeriodDuration = uint16(0);
    
    %% get the indices that should actually be presented
    movementInds = find(whichMovements);
    
    movementOrder = uint32(zeros([MAX_REPETITIONS length(find(whichMovements))]));
    numMovements = uint32(0);
    cycleNum = uint32(0);
    movementNum = uint32(0);
    currentMovement = uint32(0);
    orderSet = false;
end




%% INITIALIZE NETWORK FORMATS
if(clock < 100)
    networkOutput.discrete.send = false;
    networkOutput.continuous.send = false;
    networkOutput.screen.send = false;
    if(mod(clock, 10)==0)
        networkOutput.sendFormat = true;
    else
        networkOutput.sendFormat = false;
    end
    pauseTriggered = true; % Don't run state machine for the first 100 ms
    stateTimer = 0;
else
    networkOutput.discrete.send = false;
    networkOutput.continuous.send = true;
    networkOutput.neural.send = true;
    networkOutput.screen.send = true;
    networkOutput.sound.send = false;
    networkOutput.sendFormat = false;
end


%% ALWAYS PARSE BEHAVIOR PACKETS IF THERE ARE ANY
if(laptopPacketLength == 528)
    behaviorPacket = parseBehaviorPacket(laptopPacketData);
end

if(vizPacketLength >0)
    vizPacket = parseVizPacket(vizPacketData);
end


INIT_LENGTH = 100; %ms
PRE_MOVE_LENGTH = 10; %ms
MOVEMENT_TEXT = char(zeros([1 50]));
GO_CUE_TEXT = ['Go' char(zeros([1 48]))];
HOLD_CUE_TEXT = ['Hold' char(zeros([1 46]))];
RETURN_CUE_TEXT = ['Return' char(zeros([1 44]))];
REST_CUE_TEXT = ['Rest' char(zeros([1 46]))];

%% STATE MACHINE
switch state
    case {MovementStates.STATE_INIT}
        movementText = char(zeros([1 50]));
        networkOutput.discrete.send = false;
        %% set all the persistents that may have been changed by user input
        movementDuration = movementCueingParameters.movementDuration;
        holdDuration = movementCueingParameters.holdDuration;
        restDuration = movementCueingParameters.restDuration;
        returnDuration = movementCueingParameters.returnDuration;
        repsPerBlock = movementCueingParameters.repsPerBlock;
        randomSeed = movementCueingParameters.randomSeed;
        whichMovements = movementCueingParameters.whichMovements;
        useRandomDelay = movementCueingParameters.useRandomDelay;
        
        expRandMu = movementCueingParameters.expRandMu;
        expRandMin = movementCueingParameters.expRandMin;
        expRandMax = movementCueingParameters.expRandMax;
        expRandBinSize = movementCueingParameters.expRandBinSize;

        %pauseTriggered = stateParameters.pause;
        if behaviorPacket.mouse(6)
            pauseTriggered = false;
        end
        
        %% add entropy
        jnk = rand(1);
        
        if ~pauseTriggered
            stateTimer = stateTimer + 1;
        end
        if stateTimer >= INIT_LENGTH
            state = uint16(MovementStates.STATE_PRE_MOVE);
            stateTimer = 0;
            networkOutput.discrete.send = true;
            
            movementInds = find(whichMovements);
            numMovements = uint32(length(find(whichMovements)));
            
            cycleNum = uint32(1);
            movementNum = uint32(1);
            
            if ~orderSet
                % initialize the random ordering for the first time
                for nx = 1:repsPerBlock
                    movementOrder(nx,:) = movementInds(randperm(numMovements));
                end
                orderSet = true;
            end
            
        end
    case {MovementStates.STATE_PRE_MOVE}
        movementText = char(zeros([1 50]));
        %pauseTriggered = stateParameters.pause;
        if ~pauseTriggered
            stateTimer = stateTimer + 1;
        end
        if stateTimer >= PRE_MOVE_LENGTH
            currentMovement = movementOrder(cycleNum, movementNum);
            state = uint16(MovementStates.STATE_MOVEMENT_TEXT);
            stateTimer = 0;
            networkOutput.discrete.send = true;
            if useRandomDelay
                %% pick a new random delay
                delayPeriodDuration = uint16(0);
                while double(delayPeriodDuration) < expRandMin || double(delayPeriodDuration) > expRandMax
                     delayPeriodDuration = uint16(expRandMu * -log(rand([1 1])));
                end
                delayPeriodDuration = uint16(round(double(delayPeriodDuration) / double(expRandBinSize))*expRandBinSize);
            else
                delayPeriodDuration = uint16(expRandMu);
            end
        end
    case {MovementStates.STATE_MOVEMENT_TEXT}
        movementText = getMovementText(currentMovement);
        networkOutput.discrete.send = false;
        stateTimer = stateTimer + 1;
        if stateTimer >= delayPeriodDuration
            state = uint16(MovementStates.STATE_GO_CUE);
            stateTimer = 0;
            networkOutput.discrete.send = true;
        end
    case {MovementStates.STATE_GO_CUE}
        movementText = GO_CUE_TEXT;
        networkOutput.discrete.send = false;
        stateTimer = stateTimer + 1;
        if stateTimer >= movementDuration
            state = uint16(MovementStates.STATE_HOLD_CUE);
            stateTimer = 0;
            networkOutput.discrete.send = true;
        end
        
    case {MovementStates.STATE_HOLD_CUE}
        movementText = HOLD_CUE_TEXT;
        networkOutput.discrete.send = false;
        stateTimer = stateTimer + 1;
        if stateTimer >= holdDuration
            state = uint16(MovementStates.STATE_RETURN_CUE);
            stateTimer = 0;
            networkOutput.discrete.send = true;
        end
        
    case {MovementStates.STATE_RETURN_CUE}
        movementText = RETURN_CUE_TEXT;
        networkOutput.discrete.send = false;
        stateTimer = stateTimer + 1;
        if stateTimer >= returnDuration
            state = uint16(MovementStates.STATE_REST_CUE);
            stateTimer = 0;
            networkOutput.discrete.send = true;
        end
        
    case {MovementStates.STATE_REST_CUE}
        movementText = REST_CUE_TEXT;
        networkOutput.discrete.send = false;
        stateTimer = stateTimer + 1;
        if stateTimer >= restDuration
            stateTimer = 0;
            networkOutput.discrete.send = true;
            movementNum = movementNum +1;
            state = uint16(MovementStates.STATE_PRE_MOVE);

            if movementNum > length(movementInds)
                movementNum = uint32(1);
                cycleNum = cycleNum+1;
            end    
            
            if cycleNum > repsPerBlock
                state = uint16(MovementStates.STATE_END);
            end
        end
    
    case {MovementStates.STATE_END}
        networkOutput.discrete.send = false;
        stateTimer = stateTimer + 1;
                
end

%% PACK DATA FOR UDP OUTPUT

[networkOutput.continuous.data, networkOutput.continuous.dataLen, networkOutput.continuous.format, networkOutput.continuous.formatLen] = packDataAndFormat( ...
    TASK_NAME, VERSION_ID, ...
    'clock', clock, ...
    'xpcRequestClock', behaviorPacket.xpcRequestClock, ...
    'state', state, ...
    'currentMovement', currentMovement, ...
    'imuAngle', behaviorPacket.imuAngle, ...
    'imuAccel', behaviorPacket.imuAccel, ...
    'imuGyro', behaviorPacket.imuGyro, ...
    'imuCompass', behaviorPacket.imuCompass, ...
    'imuDataAge', behaviorPacket.imuDataAge, ...
    'glove', behaviorPacket.glove, ...
    'gloveDataAge', behaviorPacket.gloveDataAge, ...
    'mouse', behaviorPacket.mouse, ...
    'laptopTimeStamp', behaviorPacket.laptopTimestamp,...
    'xpcScreenUpdateClock',vizPacket.xpcScreenUpdateClock, ...
    'minSpikeBand', processedNeural.minSpikeBand, ...
    'minSpikeBandInd', processedNeural.minSpikeBandInd, ...
    'maxSpikeBand', processedNeural.maxSpikeBand, ...
    'maxSpikeBandInd', processedNeural.maxSpikeBandInd, ...
    'meanSquared', processedNeural.meanSquared, ...
    'meanSquaredChannel', processedNeural.meanSquaredChannel, ...
    'numDroppedUDPPackets', processedNeural.numDroppedUDPPackets ...
    );

%% SEND DISCRETE DATA TO FILELOGGER
[networkOutput.discrete.data, networkOutput.discrete.dataLen, networkOutput.discrete.format, networkOutput.discrete.formatLen] = packDataAndFormat( ...
    TASK_NAME, VERSION_ID, ...
    'clock', clock,...
    'state', state, ...
    'delayPeriodDuration', delayPeriodDuration, ...
    'useRandomDelay', useRandomDelay, ...
    'expRandMu', expRandMu, ...
    'expRandMin', expRandMin, ...
    'expRandMax', expRandMax, ...
    'expRandBinSize', expRandBinSize, ...
    'movementDuration', movementDuration, ...
    'holdDuration', holdDuration, ...
    'restDuration', restDuration, ...
    'repsPerBlock', repsPerBlock, ...
    'randomSeed', randomSeed, ...
    'whichMovements', whichMovements, ...
    'cycleNum', cycleNum, ...
    'movementNum', movementNum ...
    );

%% NEURAL DATA FOR UDP OUTPUT
[networkOutput.neural.data, networkOutput.neural.dataLen, networkOutput.neural.format, networkOutput.neural.formatLen] = packDataAndFormat( ...
    TASK_NAME, VERSION_ID, ...
    'clock', clock, ...
    'cerebusFrame',cerebusFrame(:,1),...
    'xpcTET', single(xpcTET), ...
    'outputValid', processedNeural.outputValid ...
    );

    
%% SEND DATA OUT TO VIZ
[networkOutput.screen.data, networkOutput.screen.dataLen, networkOutput.screen.format,  networkOutput.screen.formatLen] = packDataAndFormat( ...
    TASK_NAME, VERSION_ID, ...
    'clock', clock,...
    'state',state,...
    'movementText',movementText ...
    ); 


end

function behaviorPacket = parseBehaviorPacket(packetData)

    behaviorPacket.xpcRequestClock = typecast(packetData(28+[1:4]), 'uint32');
    behaviorPacket.imuAngle = typecast(packetData(32+[1:12]), 'single');
    behaviorPacket.imuAccel = typecast(packetData(44+[1:12]), 'single');
    behaviorPacket.imuGyro = typecast(packetData(56+[1:12]), 'single');
    behaviorPacket.imuCompass = typecast(packetData(68+[1:12]), 'single');
    behaviorPacket.imuDataAge = typecast(packetData(80+[1:4]), 'single');
    behaviorPacket.glove = typecast(packetData(84+[1:10]), 'uint16');
    behaviorPacket.gloveDataAge = typecast(packetData(94+[1:4]), 'single');
    behaviorPacket.mouse = typecast(packetData(98+[1:24]), 'int32');
    behaviorPacket.laptopTimestamp = typecast(packetData(122+[1:16]), 'uint8');

end


function behaviorPacket = initBehaviorPacket()

    behaviorPacket.xpcRequestClock = uint32(0);
    behaviorPacket.imuAngle = single(zeros(3,1));
    behaviorPacket.imuAccel = single(zeros(3,1));
    behaviorPacket.imuGyro = single(zeros(3,1));
    behaviorPacket.imuCompass = single(zeros(3,1));
    behaviorPacket.imuDataAge = single(inf);
    behaviorPacket.glove = uint16(zeros(5,1));
    behaviorPacket.gloveDataAge = single(inf);
    behaviorPacket.mouse = int32(zeros(6,1));
    behaviorPacket.laptopTimestamp = uint8(zeros(16,1));

end

function vizPacket = parseVizPacket(packetData)

    vizPacket.xpcScreenUpdateClock = typecast(packetData(28+[1:4]), 'uint32');

end

function vizPacket = initVizPacket()

    vizPacket.xpcScreenUpdateClock = uint32(0);

end


function retVal2 = getMovementText(moveType)
retVal2 = char(zeros([1 50]));
switch moveType
    case movementTypes.FIST
        retVal = 'Prepare: Fist';
    case movementTypes.THUMB
        retVal = 'Prepare: Thumb';
    case movementTypes.INDEX
        retVal = 'Prepare: Index';
    case movementTypes.MIDDLE
        retVal = 'Prepare: Middle';
    case movementTypes.RING
        retVal = 'Prepare: Ring';
    case movementTypes.WRISTFLEX
        retVal = 'Prepare: Wrist Flexion';
    case movementTypes.WRISTROT
        retVal = 'Prepare: Wrist Rotation';
    case movementTypes.ELBOWFLEX
        retVal = 'Prepare: Elbow';
    case movementTypes.HUMERALIN
        retVal = 'Prepare: Forearm In';
    case movementTypes.ULNAR
        retVal = 'Prepare: Ulnar Deviation';
    otherwise
        retVal = char(zeros([1 50]));
end

retVal2(1:length(retVal)) = retVal;
end

== matlab function movementCueEast/Cerebus Parallel/cerebus Parallel ==
  data: clock input uint32 size=1; digitalOut output double size=1; blockNumber input uint32 size=1
function digitalOut = digitalCerebusData(clock, blockNumber)
%#codegen
persistent digitalFrame

zeroOne = uint32(1431655765); % the bits of this number alternate between 0 and 1

if(isempty(digitalFrame))
    digitalFrame = uint32([zeroOne zeroOne uint32(blockNumber) uint32(clock) zeroOne zeroOne]);
end

frameLengthBits = 32*length(digitalFrame); % number of bits in the frame

bitPosition = mod(clock, frameLengthBits); % what position are we in for frame output

if(bitPosition==0) % if we are position zero, setup a new frame
    digitalFrame = uint32([zeroOne zeroOne blockNumber clock zeroOne zeroOne]);
end


arrayPosition = floor(double(bitPosition)/32) + 1; % which int32 of the frame are we outputting?
outputInteger = digitalFrame(arrayPosition);

digitalOut = double( bitget(outputInteger, mod(bitPosition,32) + 1) ); % which bit of that int32?

== matlab function movementCueEast/request data from laptop/Laptop Data Request ==
  data: clock input uint32 size=1; send output; data output; dataLen output
function [send, data, dataLen] = laptopDataRequest(clock)
%#codegen

data = uint8(zeros(1, 500));
data(1:4) = typecast(clock, 'uint8');
dataLen = uint16(length(data));

% Transmit 12 serial bytes every 100 ms
if(mod(clock, 10)==0)
    send = true;
else
    send = false;
end

send = true;
